simulink model "controle_espaco_estados_zr_de_0_002"  (R2015a)
settings: Solver=ode23t  StartTime=0.0  StopTime=10.0  RelTol=1e-3
settings Model: Creator=Joacy Mesquita  LastModifiedBy=Joacy Mesquita

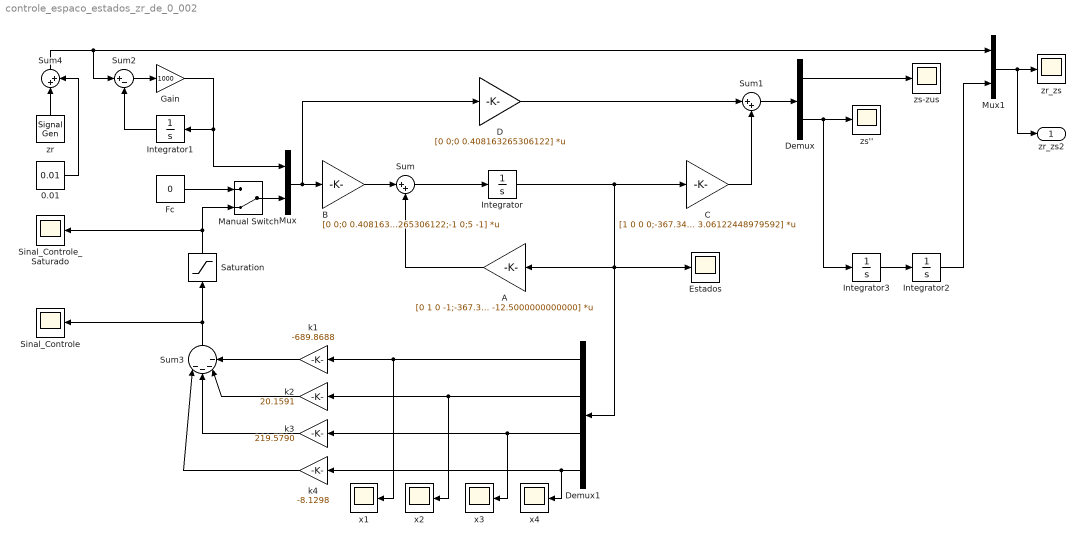
== system controle_espaco_estados_zr_de_0_002 ==
  0.01 : Constant  Value=0.01
  A : Gain  Gain=[0 1 0 -1;-367.346938775510 -3.06122448979592 0 3.06122448979592;0 0 0 1;900 7.50000000000000 -1250 -12.5000000000000]  Multiplication=Matrix(K*u)
  B : Gain  Gain=[0 0;0 0.408163265306122;-1 0;5 -1]  Multiplication=Matrix(K*u)
  C : Gain  Gain=[1 0 0 0;-367.346938775510 -3.06122448979592 0 3.06122448979592]  Multiplication=Matrix(K*u)
  D : Gain  Gain=[0 0;0 0.408163265306122]  Multiplication=Matrix(K*u)
  Demux : Demux  Outputs=2
  Demux1 : Demux
  Estados : Scope
  Fc : Constant  Value=0
  Gain : Gain  Gain=1000
  Integrator{,1..3} (4 alike) : Integrator
  Manual Switch : ManualSwitch  CurrentSetting=0
  Mux : Mux  Inputs=2
  Mux1 : Mux  Inputs=2
  Saturation : Saturate  UpperLimit=30  LowerLimit=-30
  Sinal_Controle : Scope
      settings: SaveName=ScopeData7
  Sinal_Controle_Saturado : Scope
      settings: SaveName=ScopeData8
  Sum : Sum  Inputs=|++
  Sum1 : Sum  Inputs=|++
  Sum2 : Sum  Inputs=|+-
  Sum3 : Sum  Inputs=|----
  Sum4 : Sum  Inputs=|++
  k1 : Gain  Gain=-689.8688
  k2 : Gain  Gain=20.1591
  k3 : Gain  Gain=219.5790
  k4 : Gain  Gain=-8.1298
  x{1..4} (4 alike) : Scope
      x1 settings: SaveName=ScopeData2
      x2 settings: SaveName=ScopeData3
      x3 settings: SaveName=ScopeData4
      x4 settings: SaveName=ScopeData5
  zr : SignalGenerator  WaveForm=square  Amplitude=-0.01  Frequency=0.3
  zr_zs : Scope
      settings: SaveName=ScopeData6
  zs'' : Scope
      settings: SaveName=ScopeData10
  zs-zus : Scope
      settings: SaveName=ScopeData9
  zr_zs2 : Outport
  wires:
  Mux/1 -> B/1, D/1
  B/1 -> Sum/1
  Sum/1 -> Integrator/1
  Integrator/1 -> C/1, Estados/1, Demux1/1, A/1
  D/1 -> Sum1/1
  C/1 -> Sum1/2
  Sum4/1 -> Sum2/1, Mux1/1
  Gain/1 -> Mux/1, Integrator1/1
  Sum2/1 -> Gain/1
  Integrator1/1 -> Sum2/2
  Sum1/1 -> Demux/1
  Demux1/1 -> x1/1, k1/1
  Demux1/2 -> x2/1, k2/1
  Demux1/3 -> x3/1, k3/1
  Integrator3/1 -> Integrator2/1
  Demux/2 -> Integrator3/1, zs''/1
  Integrator2/1 -> Mux1/2
  Mux1/1 -> zr_zs2/1, zr_zs/1
  Demux/1 -> zs-zus/1
  Manual Switch/1 -> Mux/2
  Fc/1 -> Manual Switch/1
  k1/1 -> Sum3/4
  k2/1 -> Sum3/3
  k3/1 -> Sum3/2
  Sum3/1 -> Saturation/1, Sinal_Controle/1
  A/1 -> Sum/2
  Demux1/4 -> x4/1, k4/1
  Saturation/1 -> Sinal_Controle_Saturado/1, Manual Switch/2
  k4/1 -> Sum3/1
  zr/1 -> Sum4/1
  0.01/1 -> Sum4/2
